simulink model "peacockElettricaSimulink"  (R2026a)
settings: Solver=FixedStepAuto  StopTime=40  FixedStep=0.001  EnableMultiTasking=on
InitFcn:
  | run('setupParams.m');
  | %run("tracks\track2.m");
StopFcn:
  | plot(out.X, out.Y);
  | axis equal;
  | grid on;
model workspace: external: MATLAB File (data not in the file)
values from neighbouring files (symbols this model uses):
  aero_bal_r = 0.5    [setupParams.m]    (also in setupParamsSingle.m)
  Af = 1.1    [setupParams.m]    (also in setupParamsSingle.m)
  auto_speed = 0    [setupParams.m]
  ay_limit = 15.0    (= 15)    [setupParams.m]    (also in setupParamsSingle.m)
  brake_bias_f = 0.40    (= 0.4)    [setupParams.m]    (also in setupParamsSingle.m = 0.6)
  brake_bias_r = 1 - brake_bias_f    (= 0.6)    [setupParams.m]    (also in setupParamsSingle.m = 0.4)
  camber_front = -1.5    [setupParams.m]    (also in setupParamsSingle.m)
  camber_rear = -1    [setupParams.m]    (also in setupParamsSingle.m)
  Cl = 1.0    (= 1)    [setupParams.m]    (also in setupParamsSingle.m)
  deathzone_APP = 5    [setupParams.m]    (also in setupParamsSingle.m)
  e_yaw_deadzone = 0.03    [setupParams.m]
  falling_slew_rate_torque = -500    [setupParams.m]    (also in setupParamsSingle.m)
  g = 9.81    [setupParams.m]    (also in setupParamsSingle.m)
  gnd_displ = 0.0    (= 0)    [setupParams.m]    (also in setupParamsSingle.m)
  h_o = 0.35    [setupParams.m]    (also in setupParamsSingle.m)
  I_charge_max = 21    [setupParams.m]
  I_discharge_max = 90    [setupParams.m]
  K_roll_rear = 0.6    [setupParams.m]    (also in setupParamsSingle.m = 0.5)
  Kus = 0.03    [setupParams.m]    (also in setupParamsSingle.m = 0)
  l_f = 0.775    [setupParams.m]    (also in setupParamsSingle.m)
  l_r = 0.775    [setupParams.m]    (also in setupParamsSingle.m)
  launch_ramp_rate = 1000.0    (= 1000)    [setupParams.m]    (also in setupParamsSingle.m)
  launch_V_thresh = 5.0    (= 5)    [setupParams.m]    (also in setupParamsSingle.m)
  mass = 320    [setupParams.m]    (also in setupParamsSingle.m = 300)
  mu = 1.5    [setupParams.m]    (also in setupParamsSingle.m)
  nominal_ramp_rate = 1000.0    (= 1000)    [setupParams.m]    (also in setupParamsSingle.m)
  overslip_factor = 1.01    [setupParams.m]    (also in setupParamsSingle.m = 1.13)
  pa_front_wheel = 82700    [setupParams.m]    (also in setupParamsSingle.m)
  pa_rear_wheel = 82700    [setupParams.m]    (also in setupParamsSingle.m)
  pedal_bp = (0:10:100)'    [setupParams.m]    (also in setupParamsSingle.m)
  pedal_map = (pedal_bp / 100) .^ pedal_alpha    [setupParams.m]    (also in setupParamsSingle.m = (pedal_bp / 100) .^ pedal_alpha.Value)
  R_wheel = 0.2032    [setupParams.m]    (also in setupParamsSingle.m)
  regen_I_cont_A = 14.0    (= 14)    [setupParams.m]    (also in setupParamsSingle.m)
  regen_I_peak_A = 21.0    (= 21)    [setupParams.m]    (also in setupParamsSingle.m)
  regen_I_peak_dur_s = 4.0    (= 4)    [setupParams.m]    (also in setupParamsSingle.m)
  regen_P_batt_max_W = 35000    [setupParams.m]    (also in setupParamsSingle.m)
  regen_pedal_thr = 5.0    (= 5)    [setupParams.m]    (also in setupParamsSingle.m = 10)
  regen_speed_crit_rpm = 1000    [setupParams.m]    (also in setupParamsSingle.m = 500)
  regen_speed_min_rpm = 4000    [setupParams.m]    (also in setupParamsSingle.m = 3000)
  regen_T_max = 9    [setupParams.m]    (also in setupParamsSingle.m = Simulink.Parameter(T_rated.Value/2))
  rho = 1.225    [setupParams.m]    (also in setupParamsSingle.m)
  rid_eff = 0.80    (= 0.8)    [setupParams.m]    (also in setupParamsSingle.m)
  rid_ratio = 15    [setupParams.m]    (also in setupParamsSingle.m)
  rising_slew_rate_torque = 100    [setupParams.m]    (also in setupParamsSingle.m)
  rpm_safe_threshold = 100    [setupParams.m]
  scale_factor_front = ones(27, 1)    [setupParams.m]    (also in setupParamsSingle.m)
  scale_factor_rear = ones(27, 1)    [setupParams.m]    (also in setupParamsSingle.m)
  slip_bc_coeff = 10    [setupParams.m]    (also in setupParamsSingle.m = Simulink.Parameter(1.5))
  slip_filt_N = 80    [setupParams.m]    (also in setupParamsSingle.m = 15)
  slip_Kd = 0.8    [setupParams.m]    (also in setupParamsSingle.m = Simulink.Parameter(5.0))
  slip_Ki = 13.0    (= 13)    [setupParams.m]    (also in setupParamsSingle.m = Simulink.Parameter(110.0))
  slip_Kp = 50.0    (= 50)    [setupParams.m]    (also in setupParamsSingle.m = Simulink.Parameter(180.0))
  slip_low_sat = 0.0    (= 0)    [setupParams.m]    (also in setupParamsSingle.m)
  slip_ref = 0.15    [setupParams.m]    (also in setupParamsSingle.m = Simulink.Parameter(0.15))
  slip_up_sat = 25    [setupParams.m]    (also in setupParamsSingle.m = 21)
  slip_V_min = 3    [setupParams.m]    (also in setupParamsSingle.m = 1)
  steer_ratio = 4.2    [pure_pursuit.m]    (also in setupParams.m; setupParamsSingle.m)
  steering_deadband = 1    [setupParams.m]
  T_headroom_k = 13.0    (= 13)    [setupParams.m]    (also in setupParamsSingle.m = Simulink.Parameter(5.0))
  T_headroom_max = 9    [setupParams.m]    (also in setupParamsSingle.m = Simulink.Parameter(5.0))
  T_peak = 20    [setupParams.m]    (also in setupParamsSingle.m = 21)
  T_rated = 9.8    [setupParams.m]    (also in setupParamsSingle.m = Simulink.Parameter(9.8))
  track_width = (track_width_r + track_width_f)/2    (= 1.2)    [setupParams.m]    (also in setupParamsSingle.m = sqrt(track_width_r^2 + track_width_f^2))
  track_width_f = 1.2    [setupParams.m]    (also in setupParamsSingle.m)
  track_width_r = 1.2    [setupParams.m]    (also in setupParamsSingle.m)
  Ts = 0.01    [setupParams.m]    (also in setupParamsSingle.m)
  tvc_bc = 17    [setupParams.m]
  tvc_D_thresh = 0.060    (= 0.06)    [setupParams.m]    (also in setupParamsSingle.m)
  tvc_D_thresh_off = 0.03    [setupParams.m]    (also in setupParamsSingle.m)
  tvc_Kd = 100    [setupParams.m]    (also in setupParamsSingle.m = Simulink.Parameter(5))
  tvc_Ki = 150    [setupParams.m]    (also in setupParamsSingle.m = Simulink.Parameter(10))
  tvc_Kp = 650    [setupParams.m]    (also in setupParamsSingle.m = Simulink.Parameter(70))
  tvc_N_filter = 25    [setupParams.m]    (also in setupParamsSingle.m = Simulink.Parameter(20))
  tvc_sat_dMz = 700    [setupParams.m]    (also in setupParamsSingle.m = Simulink.Parameter(10.0))
  tvc_throttle_on = 3.0    (= 3)    [setupParams.m]    (also in setupParamsSingle.m = Simulink.Parameter(3.0))
  tvc_tr = 5    [setupParams.m]    (also in setupParamsSingle.m = Simulink.Parameter(1.0))
  tvc_V_off = 2.0    (= 2)    [setupParams.m]    (also in setupParamsSingle.m = Simulink.Parameter(2.0))
  tvc_V_on = 4.0    (= 4)    [setupParams.m]    (also in setupParamsSingle.m = Simulink.Parameter(4.0))
  tvc_yaw_thresh = 0.08    [setupParams.m]    (also in setupParamsSingle.m)
  tvc_yaw_thresh_off = 0.04    [setupParams.m]    (also in setupParamsSingle.m)
  V_dc = 540    [setupParams.m]    (also in setupParamsSingle.m)
  w_engine = 0.005    [setupParams.m]    (also in setupParamsSingle.m)
  wheelbase = l_f + l_r    (= 1.55)    [setupParams.m]    (also in setupParamsSingle.m)
undefined symbols (not defined in the file or in its folder): V_ref, X_ref, Y_ref
libraries: simulink x74, slpidlib x8, vehdynlibtire x8, dspsigops x4, vehdynlibsteering x2, autolibshared x2, sim3dautolib x2, sim3dlib x1, robotalgslib x1
(part 3 of 6)

== system peacockElettricaSimulink/Signal Brake Builder ==
  note: TEST2
  note: TEST1
  note: TEST3
  Constant : Constant  Value=0
  Ramp1 : simulink/Sources/Ramp  slope=50  start=20  InitialOutput=0
  Ramp10 : simulink/Sources/Ramp  slope=-30  start=21  InitialOutput=0
  Ramp3 : simulink/Sources/Ramp  slope=-30  start=33.5  InitialOutput=0
  Saturation1 : Saturate  UpperLimit=50  LowerLimit=-70
  Saturation{3,5,7,11} (4 alike) : Saturate  UpperLimit=100  LowerLimit=-70
  Saturation2 : Saturate  UpperLimit=50  LowerLimit=-50
  Saturation4 : Saturate  UpperLimit=70  LowerLimit=0
  Saturation6 : Saturate  UpperLimit=100  LowerLimit=0
  Saturation8 : Saturate  UpperLimit=70  LowerLimit=0
  Step3 : Step  Time=33  FinalValue=30  SampleTime=0
  Sum1 : Sum  Inputs=|+-
  Sum2 : Sum  Inputs=|+-
  Sum3 : Sum  Inputs=|++++
  t17 : simulink/Sources/Ramp  slope=50  start=17  InitialOutput=0
  t20_2 : simulink/Sources/Ramp  slope=+50  start=20  InitialOutput=0
  t26 : simulink/Sources/Ramp  slope=50  start=26  InitialOutput=0
  t36_2 : simulink/Sources/Ramp  slope=50  start=36  InitialOutput=0
  Brake_% : Outport
  wires:
  Constant/1 -> ?
  Sum1/1 -> ?
  t17/1 -> Saturation1/1
  Saturation4/1 -> Sum3/1
  Saturation1/1 -> Sum2/1  "50%"
  Sum3/1 -> Saturation6/1
  Saturation8/1 -> Sum3/3
  Saturation6/1 -> Brake_%/1
  Ramp3/1 -> Saturation7/1
  Sum2/1 -> ?
  t26/1 -> Saturation3/1
  Saturation2/1 -> Sum2/2  "-50%"
  Saturation7/1 -> Sum3/4
  Ramp1/1 -> Saturation4/1  "80%"
  Saturation3/1 -> Sum1/1  "100%"
  t36_2/1 -> Saturation5/1
  Ramp10/1 -> Saturation11/1
  t20_2/1 -> Saturation2/1
  Saturation5/1 -> Sum1/2  "t36%"
  Saturation11/1 -> Sum3/2
  Step3/1 -> Saturation8/1  "80%"

== system peacockElettricaSimulink/Signal Brake Builder_ ==
  note: TEST2
  note: TEST1
  note: TEST3
  Constant : Constant  Value=0
  Ramp1 : simulink/Sources/Ramp  slope=50  start=20  InitialOutput=0
  Ramp10 : simulink/Sources/Ramp  slope=-30  start=21  InitialOutput=0
  Ramp3 : simulink/Sources/Ramp  slope=-30  start=33.5  InitialOutput=0
  Saturation1 : Saturate  UpperLimit=50  LowerLimit=-70
  Saturation{3,5,7,11} (4 alike) : Saturate  UpperLimit=100  LowerLimit=-70
  Saturation2 : Saturate  UpperLimit=50  LowerLimit=-50
  Saturation4 : Saturate  UpperLimit=70  LowerLimit=0
  Saturation6 : Saturate  UpperLimit=100  LowerLimit=0
  Saturation8 : Saturate  UpperLimit=70  LowerLimit=0
  Step3 : Step  Time=33  FinalValue=30  SampleTime=0
  Sum1 : Sum  Inputs=|+-
  Sum2 : Sum  Inputs=|+-
  Sum3 : Sum  Inputs=|++++
  t17 : simulink/Sources/Ramp  slope=50  start=17  InitialOutput=0
  t20_2 : simulink/Sources/Ramp  slope=+50  start=20  InitialOutput=0
  t26 : simulink/Sources/Ramp  slope=50  start=26  InitialOutput=0
  t36_2 : simulink/Sources/Ramp  slope=50  start=36  InitialOutput=0
  Brake_% : Outport
  wires:
  Constant/1 -> ?
  Sum1/1 -> ?
  t17/1 -> Saturation1/1
  Saturation4/1 -> Sum3/1
  Saturation1/1 -> Sum2/1  "50%"
  Sum3/1 -> Saturation6/1
  Saturation8/1 -> Sum3/3
  Saturation6/1 -> Brake_%/1
  Ramp3/1 -> Saturation7/1
  Sum2/1 -> ?
  t26/1 -> Saturation3/1
  Saturation2/1 -> Sum2/2  "-50%"
  Saturation7/1 -> Sum3/4
  Ramp1/1 -> Saturation4/1  "80%"
  Saturation3/1 -> Sum1/1  "100%"
  t36_2/1 -> Saturation5/1
  Ramp10/1 -> Saturation11/1
  t20_2/1 -> Saturation2/1
  Saturation5/1 -> Sum1/2  "t36%"
  Saturation11/1 -> Sum3/2
  Step3/1 -> Saturation8/1  "80%"

== system peacockElettricaSimulink/Signal Steering Builde_r ==
  note: TEST2
  note: TEST1
  Constant1 : Constant  Value=0
  Ramp : simulink/Sources/Ramp  slope=20  start=3  InitialOutput=0
  Ramp1 : simulink/Sources/Ramp  slope=-20  start=7  InitialOutput=0
  Ramp2 : simulink/Sources/Ramp  slope=-30  start=7  InitialOutput=0
  Ramp3 : simulink/Sources/Ramp  slope=20  start=11  InitialOutput=0
  Ramp4 : simulink/Sources/Ramp  slope=30  start=4  InitialOutput=0
  Ramp5 : simulink/Sources/Ramp  slope=30  start=25  InitialOutput=0
  Ramp6 : simulink/Sources/Ramp  slope=-20  start=27  InitialOutput=0
  Ramp7 : simulink/Sources/Ramp  slope=-40  start=35  InitialOutput=0
  Ramp8 : simulink/Sources/Ramp  slope=30  start=37  InitialOutput=0
  Saturation{,1..5} (6 alike) : Saturate  UpperLimit=40  LowerLimit=-40
  Saturation{8..11} (4 alike) : Saturate  UpperLimit=50  LowerLimit=-50
  Saturation6 : Saturate  UpperLimit=60  LowerLimit=-60
  Saturation7 : Saturate  UpperLimit=60  LowerLimit=-60
  Sum1 : Sum  Inputs=|++++++++
  Sum2 : Sum  Inputs=|+-+-
  t2 : simulink/Sources/Ramp  slope=20  start=2  InitialOutput=0
  t20 : simulink/Sources/Ramp  slope=-20  start=20  InitialOutput=0
  t30 : simulink/Sources/Ramp  slope=-20  start=30  InitialOutput=0
  t8 : simulink/Sources/Ramp  slope=20  start=8  InitialOutput=0
  Out1 : Outport
  wires:
  Ramp4/1 -> ?
  Constant1/1 -> ?
  Sum2/1 -> ?
  Saturation9/1 -> Sum2/2
  t30/1 -> Saturation11/1
  Ramp1/1 -> Saturation1/1
  Ramp7/1 -> Saturation6/1
  Saturation2/1 -> Sum1/3
  Saturation10/1 -> Sum2/3
  Saturation3/1 -> Sum1/4
  Ramp3/1 -> Saturation3/1
  Saturation11/1 -> Sum2/4
  Saturation7/1 -> Sum1/8
  Saturation/1 -> Sum1/1
  t2/1 -> Saturation8/1
  t20/1 -> Saturation10/1
  Ramp8/1 -> Saturation7/1
  Ramp5/1 -> Saturation4/1
  Saturation8/1 -> Sum2/1
  Saturation1/1 -> Sum1/2
  Ramp2/1 -> Saturation2/1
  t8/1 -> Saturation9/1
  Sum1/1 -> Out1/1
  Saturation5/1 -> Sum1/6
  Saturation6/1 -> Sum1/7
  Ramp/1 -> Saturation/1
  Saturation4/1 -> Sum1/5
  Ramp6/1 -> Saturation5/1

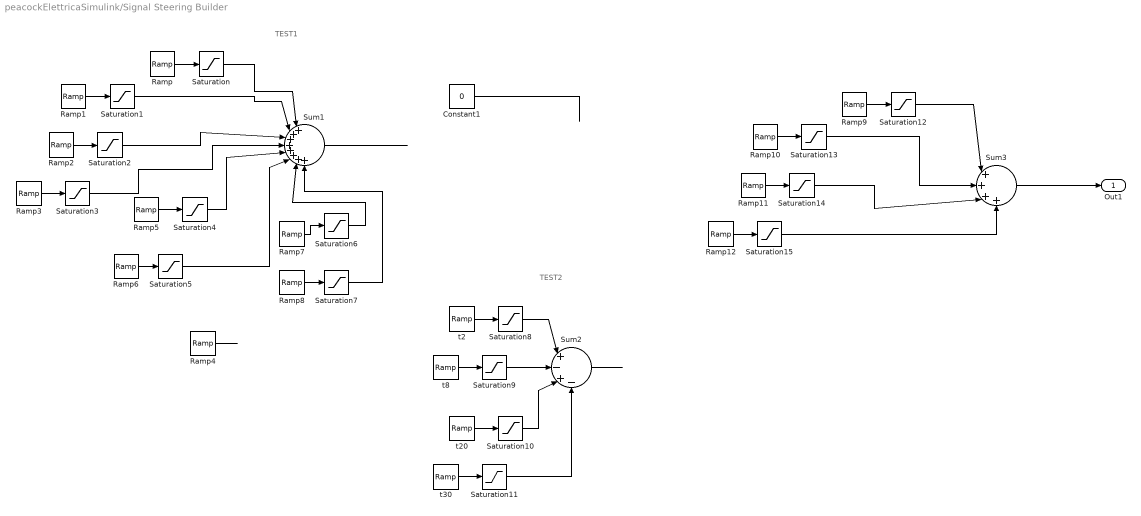
== system peacockElettricaSimulink/Signal Steering Builder ==
  note: TEST2
  note: TEST1
  Constant1 : Constant  Value=0
  Ramp : simulink/Sources/Ramp  slope=20  start=3  InitialOutput=0
  Ramp1 : simulink/Sources/Ramp  slope=-20  start=7  InitialOutput=0
  Ramp10 : simulink/Sources/Ramp  slope=-20  start=15  InitialOutput=0
  Ramp11 : simulink/Sources/Ramp  slope=-30  start=22  InitialOutput=0
  Ramp12 : simulink/Sources/Ramp  slope=30  start=27  InitialOutput=0
  Ramp2 : simulink/Sources/Ramp  slope=-30  start=7  InitialOutput=0
  Ramp3 : simulink/Sources/Ramp  slope=30  start=11  InitialOutput=0
  Ramp4 : simulink/Sources/Ramp  slope=30  start=4  InitialOutput=0
  Ramp5 : simulink/Sources/Ramp  slope=30  start=25  InitialOutput=0
  Ramp6 : simulink/Sources/Ramp  slope=-20  start=27  InitialOutput=0
  Ramp7 : simulink/Sources/Ramp  slope=-40  start=35  InitialOutput=0
  Ramp8 : simulink/Sources/Ramp  slope=30  start=37  InitialOutput=0
  Ramp9 : simulink/Sources/Ramp  slope=20  start=10  InitialOutput=0
  Saturation{,1..5,12..15} (10 alike) : Saturate  UpperLimit=40  LowerLimit=-40
  Saturation{8..11} (4 alike) : Saturate  UpperLimit=50  LowerLimit=-50
  Saturation6 : Saturate  UpperLimit=60  LowerLimit=-60
  Saturation7 : Saturate  UpperLimit=60  LowerLimit=-60
  Sum1 : Sum  Inputs=|++++++++
  Sum2 : Sum  Inputs=|+-+-
  Sum3 : Sum  Inputs=|++++
  t2 : simulink/Sources/Ramp  slope=20  start=2  InitialOutput=0
  t20 : simulink/Sources/Ramp  slope=-20  start=20  InitialOutput=0
  t30 : simulink/Sources/Ramp  slope=-20  start=30  InitialOutput=0
  t8 : simulink/Sources/Ramp  slope=20  start=8  InitialOutput=0
  Out1 : Outport
  wires:
  Ramp4/1 -> ?
  Constant1/1 -> ?
  Sum2/1 -> ?
  Saturation9/1 -> Sum2/2
  t30/1 -> Saturation11/1
  Ramp1/1 -> Saturation1/1
  Ramp7/1 -> Saturation6/1
  Saturation2/1 -> Sum1/3
  Saturation10/1 -> Sum2/3
  Saturation3/1 -> Sum1/4
  Ramp3/1 -> Saturation3/1
  Saturation11/1 -> Sum2/4
  Saturation7/1 -> Sum1/8
  Saturation/1 -> Sum1/1
  t2/1 -> Saturation8/1
  t20/1 -> Saturation10/1
  Ramp8/1 -> Saturation7/1
  Ramp5/1 -> Saturation4/1
  Saturation8/1 -> Sum2/1
  Saturation1/1 -> Sum1/2
  Ramp2/1 -> Saturation2/1
  t8/1 -> Saturation9/1
  Sum1/1 -> ?
  Saturation5/1 -> Sum1/6
  Saturation6/1 -> Sum1/7
  Ramp/1 -> Saturation/1
  Saturation4/1 -> Sum1/5
  Ramp6/1 -> Saturation5/1
  Sum3/1 -> Out1/1
  Saturation12/1 -> Sum3/1
  Saturation15/1 -> Sum3/4
  Ramp12/1 -> Saturation15/1
  Saturation13/1 -> Sum3/2
  Ramp10/1 -> Saturation13/1
  Ramp11/1 -> Saturation14/1
  Ramp9/1 -> Saturation12/1
  Saturation14/1 -> Sum3/3

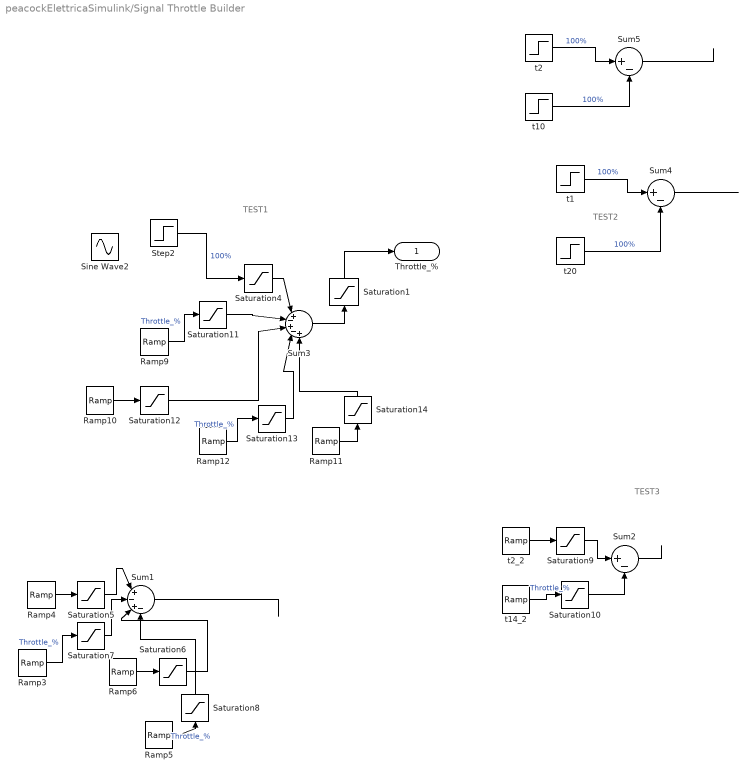
== system peacockElettricaSimulink/Signal Throttle Builder ==
  note: TEST1
  note: TEST2
  note: TEST3
  Ramp10 : simulink/Sources/Ramp  slope=50  start=26  InitialOutput=0
  Ramp11 : simulink/Sources/Ramp  slope=12  start=34  InitialOutput=0
  Ramp12 : simulink/Sources/Ramp  slope=100  start=31  InitialOutput=0
  Ramp3 : simulink/Sources/Ramp  slope=50  start=8  InitialOutput=0
  Ramp4 : simulink/Sources/Ramp  slope=150  start=1  InitialOutput=0
  Ramp5 : simulink/Sources/Ramp  slope=100  start=20  InitialOutput=0
  Ramp6 : simulink/Sources/Ramp  slope=50  start=12  InitialOutput=0
  Ramp9 : simulink/Sources/Ramp  slope=100  start=19  InitialOutput=0
  Saturation1 : Saturate  UpperLimit=50  LowerLimit=0
  Saturation{4..14} (11 alike) : Saturate  UpperLimit=100  LowerLimit=0
  Sine Wave2 : Sin  Amplitude=800  Frequency=0.3  SampleTime=Ts
  Step2 : Step  Time=2  FinalValue=100  SampleTime=0
  Sum1 : Sum  Inputs=|+-+-
  Sum2 : Sum  Inputs=|+-
  Sum3 : Sum  Inputs=|+-+-+
  Sum4 : Sum  Inputs=|+-
  Sum5 : Sum  Inputs=|+-
  t1 : Step  FinalValue=100  SampleTime=0
  t10 : Step  Time=10  FinalValue=100  SampleTime=0
  t14_2 : simulink/Sources/Ramp  slope=50  start=14  InitialOutput=0
  t2 : Step  FinalValue=100  SampleTime=0
  t20 : Step  Time=20  FinalValue=100  SampleTime=0
  t2_2 : simulink/Sources/Ramp  slope=50  start=2  InitialOutput=0
  Throttle_% : Outport
  wires:
  Sum4/1 -> ?
  Sum1/1 -> ?
  Sum2/1 -> ?
  Sum5/1 -> ?
  Step2/1 -> Saturation4/1  "100%"
  Ramp10/1 -> Saturation12/1
  Saturation7/1 -> Sum1/2
  Saturation13/1 -> Sum3/4
  Ramp9/1 -> Saturation11/1  "Throttle_%"
  t10/1 -> Sum5/2  "100%"
  Saturation5/1 -> Sum1/1
  Ramp6/1 -> Saturation6/1
  Saturation9/1 -> Sum2/1
  t2_2/1 -> Saturation9/1
  Saturation14/1 -> Sum3/5
  Saturation10/1 -> Sum2/2
  Saturation8/1 -> Sum1/4
  Saturation6/1 -> Sum1/3
  t1/1 -> Sum4/1  "100%"
  Ramp5/1 -> Saturation8/1  "Throttle_%"
  Sum3/1 -> Saturation1/1
  Ramp3/1 -> Saturation7/1  "Throttle_%"
  t20/1 -> Sum4/2  "100%"
  t2/1 -> Sum5/1  "100%"
  Ramp4/1 -> Saturation5/1
  Saturation11/1 -> Sum3/2
  Ramp12/1 -> Saturation13/1  "Throttle_%"
  Ramp11/1 -> Saturation14/1
  t14_2/1 -> Saturation10/1  "Throttle_%"
  Saturation12/1 -> Sum3/3
  Saturation4/1 -> Sum3/1
  Saturation1/1 -> Throttle_%/1

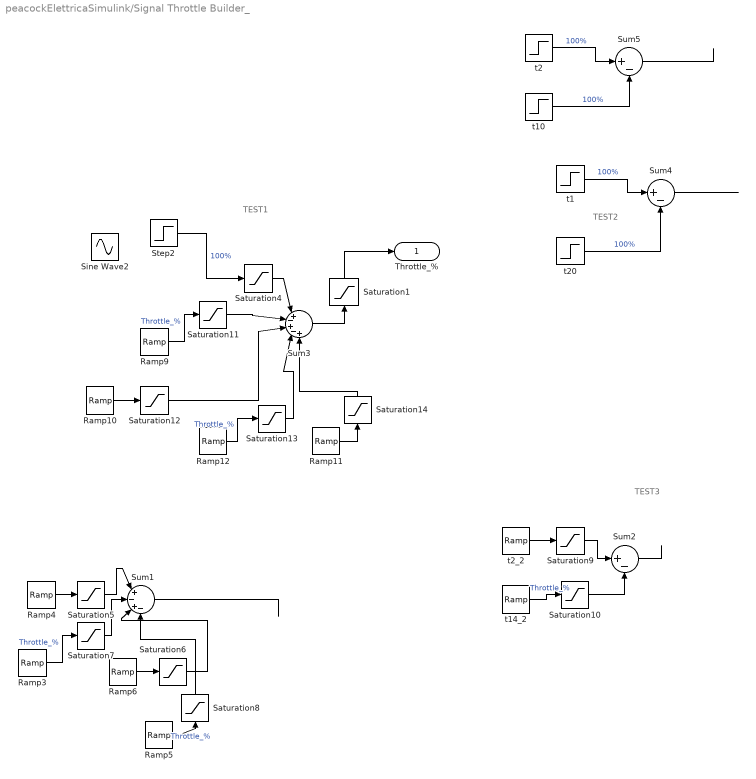
== system peacockElettricaSimulink/Signal Throttle Builder_ ==
  note: TEST1
  note: TEST2
  note: TEST3
  Ramp10 : simulink/Sources/Ramp  slope=50  start=26  InitialOutput=0
  Ramp11 : simulink/Sources/Ramp  slope=12  start=34  InitialOutput=0
  Ramp12 : simulink/Sources/Ramp  slope=100  start=31  InitialOutput=0
  Ramp3 : simulink/Sources/Ramp  slope=50  start=8  InitialOutput=0
  Ramp4 : simulink/Sources/Ramp  slope=150  start=1  InitialOutput=0
  Ramp5 : simulink/Sources/Ramp  slope=100  start=20  InitialOutput=0
  Ramp6 : simulink/Sources/Ramp  slope=50  start=12  InitialOutput=0
  Ramp9 : simulink/Sources/Ramp  slope=100  start=19  InitialOutput=0
  Saturation1 : Saturate  UpperLimit=50  LowerLimit=0
  Saturation{4..14} (11 alike) : Saturate  UpperLimit=100  LowerLimit=0
  Sine Wave2 : Sin  Amplitude=800  Frequency=0.3  SampleTime=Ts
  Step2 : Step  Time=2  FinalValue=100  SampleTime=0
  Sum1 : Sum  Inputs=|+-+-
  Sum2 : Sum  Inputs=|+-
  Sum3 : Sum  Inputs=|+-+-+
  Sum4 : Sum  Inputs=|+-
  Sum5 : Sum  Inputs=|+-
  t1 : Step  FinalValue=100  SampleTime=0
  t10 : Step  Time=10  FinalValue=100  SampleTime=0
  t14_2 : simulink/Sources/Ramp  slope=50  start=14  InitialOutput=0
  t2 : Step  FinalValue=100  SampleTime=0
  t20 : Step  Time=20  FinalValue=100  SampleTime=0
  t2_2 : simulink/Sources/Ramp  slope=50  start=2  InitialOutput=0
  Throttle_% : Outport
  wires:
  Sum4/1 -> ?
  Sum1/1 -> ?
  Sum2/1 -> ?
  Sum5/1 -> ?
  Step2/1 -> Saturation4/1  "100%"
  Ramp10/1 -> Saturation12/1
  Saturation7/1 -> Sum1/2
  Saturation13/1 -> Sum3/4
  Ramp9/1 -> Saturation11/1  "Throttle_%"
  t10/1 -> Sum5/2  "100%"
  Saturation5/1 -> Sum1/1
  Ramp6/1 -> Saturation6/1
  Saturation9/1 -> Sum2/1
  t2_2/1 -> Saturation9/1
  Saturation14/1 -> Sum3/5
  Saturation10/1 -> Sum2/2
  Saturation8/1 -> Sum1/4
  Saturation6/1 -> Sum1/3
  t1/1 -> Sum4/1  "100%"
  Ramp5/1 -> Saturation8/1  "Throttle_%"
  Sum3/1 -> Saturation1/1
  Ramp3/1 -> Saturation7/1  "Throttle_%"
  t20/1 -> Sum4/2  "100%"
  t2/1 -> Sum5/1  "100%"
  Ramp4/1 -> Saturation5/1
  Saturation11/1 -> Sum3/2
  Ramp12/1 -> Saturation13/1  "Throttle_%"
  Ramp11/1 -> Saturation14/1
  t14_2/1 -> Saturation10/1  "Throttle_%"
  Saturation12/1 -> Sum3/3
  Saturation4/1 -> Sum3/1
  Saturation1/1 -> Throttle_%/1

== system peacockElettricaSimulink/Subsystem ==
  V_ref : Inport
  V_x : Inport  Port=2
  Gain : Gain  Gain=-1
  PID Controller : slpidlib/PID Controller  Controller=PID  Form=Parallel  TimeDomain=Discrete-time  UseExternalTs=off  SampleTime=-1  IntegratorMethod=Forward Euler  FilterMethod=Forward Euler  ControllerParametersSource=internal  P=3  I=0.2  UseKiTs=off  D=0  UseExternalDerivativeSource=off  N=100  UseFilter=on  TunerSelectOption=Transfer Function Based (PID Tuner App)  InitialConditionSource=internal  InitialConditionForIntegrator=0  InitialConditionForFilter=0  DifferentiatorICPrevScaledInput=0  ExternalReset=none  TrackingMode=off  Kt=1  LimitOutput=on  SatLimitsSource=internal  UpperSaturationLimit=100  LowerSaturationLimit=-100  LinearizeAsGain=on  AntiWindupMode=clamping  Kb=1  LimitIntegrator=off  UpperIntegratorSaturationLimit=inf  LowerIntegratorSaturationLimit=-inf  POutMin=[]  POutMax=[]  IOutMin=[]  IOutMax=[]  DOutMin=[]  DOutMax=[]  NOutMin=[]  NOutMax=[]  SumOutMin=[]  SumOutMax=[]  SaturationOutMin=[]  SaturationOutMax=[]  PParamMin=[]  PParamMax=[]  IParamMin=[]  IParamMax=[]  DParamMin=[]  DParamMax=[]  NParamMin=[]  NParamMax=[]  KbParamMin=[]  KbParamMax=[]  KtParamMin=[]  KtParamMax=[]  KbOutMin=[]  KbOutMax=[]  KtOutMin=[]  KtOutMax=[]  IntegratorOutMin=[]  IntegratorOutMax=[]  FilterOutMin=[]  FilterOutMax=[]  SumI1OutMin=[]  SumI1OutMax=[]  SumI2OutMin=[]  SumI2OutMax=[]  SumI3OutMin=[]  SumI3OutMax=[]  SumI4OutMin=[]  SumI4OutMax=[]  SumDOutMin=[]  SumDOutMax=[]  DifferentiatorOutMin=[]  DifferentiatorOutMax=[]  FilterDiffOutCoefMin=[]  FilterDiffOutCoefMax=[]  ReciprocalOutMin=[]  ReciprocalOutMax=[]  SumDenOutMin=[]  SumDenOutMax=[]  SumNumOutMin=[]  SumNumOutMax=[]  DivideOutMin=[]  DivideOutMax=[]  UdiffTsProdOutMin=[]  UdiffTsProdOutMax=[]  NTsProdOutMin=[]  NTsProdOutMax=[]  UintegralTsProdOutMin=[]  UintegralTsProdOutMax=[]  UngainTsProdOutMin=[]  UngainTsProdOutMax=[]  ClampingZeroOutDataTypeStr=Inherit: Inherit via back propagation  ClampingZeroOutMin=[]  ClampingZeroOutMax=[]  FilterDenConstantOutDataTypeStr=Inherit: Inherit via back propagation  FilterDenConstantOutMin=[]  FilterDenConstantOutMax=[]  PCopyOutDataTypeStr=Inherit: Inherit via back propagation  PCopyOutMin=[]  PCopyOutMax=[]  NCopyOutDataTypeStr=Inherit: Inherit via back propagation  NCopyOutMin=[]  NCopyOutMax=[]  IntegratorContinuousStateAttributes=''  IntegratorStateMustResolveToSignalObject=off  IntegratorRTWStateStorageClass=Auto  FilterContinuousStateAttributes=''  FilterStateMustResolveToSignalObject=off  FilterRTWStateStorageClass=Auto  ParallelPVariant=InternalParameters  IdealPVariant=Disabled  IVariant=InternalParameters  DVariant=InternalParameters  IntegratorVariant=Discrete  SatVariant=Enabled  AWVariant=DiscClampingParallel  PCopyVariant=Disabled  TRVariant=Disabled  FdbkBlocksVariant=Forward  IdealPFdbkVariant=Disabled  SatFdbkVariant=Disabled  DerivativeFilterVariant=ForwardEulerFilter  NVariant=InternalParameters  NCopyVariant=Disabled  FilterICVariant=InternalICsFilter  IntegratorICVariant=InternalICs  ExternalResetVariant=Disabled  TRSumVariant=Passthrough  SumFdbkVariant=Disabled  SumVariant=Sum_PID  TsampFilterVariant=InternalTs  TsampNgainVariant=Passthrough  TsampIntegralVariant=Disabled_SignalSpec  ExternalSaturationOutDataTypeStr=Inherit: Same as second input  DerivativeSourceVariant=ErrorSignal  PreIntVariant=InternalPreInt
  Rate Limiter : RateLimiter  RisingSlewLimit=200  FallingSlewLimit=-500  SampleTimeMode=inherited
  Rate Limiter1 : RateLimiter  RisingSlewLimit=200  FallingSlewLimit=-500  SampleTimeMode=inherited
  Sum : Sum  Inputs=|+-
  brake : Saturate  UpperLimit=60  LowerLimit=0
  throttle : Saturate  UpperLimit=60  LowerLimit=0
  Throttle_% : Outport
  Brake_% : Outport  Port=2
  wires:
  PID Controller/1 -> throttle/1, Gain/1
  V_x/1 -> Sum/2
  Sum/1 -> PID Controller/1  "e_vx"
  throttle/1 -> Rate Limiter/1
  Gain/1 -> brake/1
  brake/1 -> Rate Limiter1/1
  Rate Limiter/1 -> Throttle_%/1
  Rate Limiter1/1 -> Brake_%/1
  V_ref/1 -> Sum/1

== system peacockElettricaSimulink/Subsystem1 ==
  V_x : Inport
  V_ref : Inport  Port=2
  Gain : Gain  Gain=-1
  PID Controller : slpidlib/PID Controller  Controller=PID  Form=Parallel  TimeDomain=Discrete-time  UseExternalTs=off  SampleTime=-1  IntegratorMethod=Forward Euler  FilterMethod=Forward Euler  ControllerParametersSource=internal  P=7  I=0.8  UseKiTs=off  D=1.5  UseExternalDerivativeSource=off  N=80  UseFilter=on  TunerSelectOption=Transfer Function Based (PID Tuner App)  InitialConditionSource=internal  InitialConditionForIntegrator=0  InitialConditionForFilter=0  DifferentiatorICPrevScaledInput=0  ExternalReset=none  TrackingMode=off  Kt=1  LimitOutput=on  SatLimitsSource=internal  UpperSaturationLimit=100  LowerSaturationLimit=-100  LinearizeAsGain=on  AntiWindupMode=back-calculation  Kb=2  LimitIntegrator=off  UpperIntegratorSaturationLimit=inf  LowerIntegratorSaturationLimit=-inf  POutMin=[]  POutMax=[]  IOutMin=[]  IOutMax=[]  DOutMin=[]  DOutMax=[]  NOutMin=[]  NOutMax=[]  SumOutMin=[]  SumOutMax=[]  SaturationOutMin=[]  SaturationOutMax=[]  PParamMin=[]  PParamMax=[]  IParamMin=[]  IParamMax=[]  DParamMin=[]  DParamMax=[]  NParamMin=[]  NParamMax=[]  KbParamMin=[]  KbParamMax=[]  KtParamMin=[]  KtParamMax=[]  KbOutMin=[]  KbOutMax=[]  KtOutMin=[]  KtOutMax=[]  IntegratorOutMin=[]  IntegratorOutMax=[]  FilterOutMin=[]  FilterOutMax=[]  SumI1OutMin=[]  SumI1OutMax=[]  SumI2OutMin=[]  SumI2OutMax=[]  SumI3OutMin=[]  SumI3OutMax=[]  SumI4OutMin=[]  SumI4OutMax=[]  SumDOutMin=[]  SumDOutMax=[]  DifferentiatorOutMin=[]  DifferentiatorOutMax=[]  FilterDiffOutCoefMin=[]  FilterDiffOutCoefMax=[]  ReciprocalOutMin=[]  ReciprocalOutMax=[]  SumDenOutMin=[]  SumDenOutMax=[]  SumNumOutMin=[]  SumNumOutMax=[]  DivideOutMin=[]  DivideOutMax=[]  UdiffTsProdOutMin=[]  UdiffTsProdOutMax=[]  NTsProdOutMin=[]  NTsProdOutMax=[]  UintegralTsProdOutMin=[]  UintegralTsProdOutMax=[]  UngainTsProdOutMin=[]  UngainTsProdOutMax=[]  ClampingZeroOutDataTypeStr=Inherit: Inherit via back propagation  ClampingZeroOutMin=[]  ClampingZeroOutMax=[]  FilterDenConstantOutDataTypeStr=Inherit: Inherit via back propagation  FilterDenConstantOutMin=[]  FilterDenConstantOutMax=[]  PCopyOutDataTypeStr=Inherit: Inherit via back propagation  PCopyOutMin=[]  PCopyOutMax=[]  NCopyOutDataTypeStr=Inherit: Inherit via back propagation  NCopyOutMin=[]  NCopyOutMax=[]  IntegratorContinuousStateAttributes=''  IntegratorStateMustResolveToSignalObject=off  IntegratorRTWStateStorageClass=Auto  FilterContinuousStateAttributes=''  FilterStateMustResolveToSignalObject=off  FilterRTWStateStorageClass=Auto  ParallelPVariant=InternalParameters  IdealPVariant=Disabled  IVariant=InternalParameters  DVariant=InternalParameters  IntegratorVariant=Discrete  SatVariant=Enabled  AWVariant=BackCalculation  PCopyVariant=Disabled  TRVariant=Disabled  FdbkBlocksVariant=Forward  IdealPFdbkVariant=Disabled  SatFdbkVariant=Disabled  DerivativeFilterVariant=ForwardEulerFilter  NVariant=InternalParameters  NCopyVariant=Disabled  FilterICVariant=InternalICsFilter  IntegratorICVariant=InternalICs  ExternalResetVariant=Disabled  TRSumVariant=Passthrough  SumFdbkVariant=Disabled  SumVariant=Sum_PID  TsampFilterVariant=InternalTs  TsampNgainVariant=Passthrough  TsampIntegralVariant=Disabled_SignalSpec  ExternalSaturationOutDataTypeStr=Inherit: Same as second input  DerivativeSourceVariant=ErrorSignal  PreIntVariant=InternalPreInt
  Rate Limiter : RateLimiter  RisingSlewLimit=200  FallingSlewLimit=-500  SampleTimeMode=inherited
  Rate Limiter1 : RateLimiter  RisingSlewLimit=200  FallingSlewLimit=-500  SampleTimeMode=inherited
  Sum : Sum  Inputs=|+-
  brake : Saturate  UpperLimit=60  LowerLimit=0
  throttle : Saturate  UpperLimit=100  LowerLimit=0
  Throttle_% : Outport
  Brake_% : Outport  Port=2
  wires:
  PID Controller/1 -> throttle/1, Gain/1
  V_x/1 -> Sum/2
  Sum/1 -> PID Controller/1  "e_vx"
  throttle/1 -> Rate Limiter/1
  Gain/1 -> brake/1
  brake/1 -> Rate Limiter1/1
  Rate Limiter/1 -> Throttle_%/1
  Rate Limiter1/1 -> Brake_%/1
  V_ref/1 -> Sum/1

== system peacockElettricaSimulink/DriveController/LaunchThrottleController ==
  V : Inport
  Throttle_% : Inport  Port=2
  1-D Lookup Table : Lookup_n-D  NumberOfTableDimensions=1  BreakpointsForDimension1=pedal_bp  Table=pedal_map  ExtrapMethod=Clip  UseLastTableValue=on  InternalRulePriority=Speed  RndMeth=Simplest
  Constant : Constant  Value=0
  Gain5 : Gain  Gain=100
  Rate Limiter1 : RateLimiter  RisingSlewLimit=launch_ramp_rate  FallingSlewLimit=-250  SampleTimeMode=inherited
  Rate Limiter2 : RateLimiter  RisingSlewLimit=nominal_ramp_rate  FallingSlewLimit=-250  SampleTimeMode=inherited
  Saturation : Saturate  UpperLimit=100  LowerLimit=0
  Saturation1 : Saturate  UpperLimit=100  LowerLimit=0
  Switch : Switch  Criteria=u2 > Threshold  Threshold=launch_V_thresh  SaturateOnIntegerOverflow=off  InputSameDT=off
  Switch1 : Switch  Criteria=u2 > Threshold  Threshold=deathzone_APP  SaturateOnIntegerOverflow=off  InputSameDT=off
  Throttle : Outport
  wires:
  1-D Lookup Table/1 -> Gain5/1
  Gain5/1 -> Rate Limiter1/1
  Switch1/1 -> Throttle/1  "Throttle%"
  Saturation1/1 -> Rate Limiter2/1, 1-D Lookup Table/1
  Rate Limiter2/1 -> Switch/3  "Throttle%"
  Rate Limiter1/1 -> Switch/1  "Throttle%"
  V/1 -> Switch/2
  Switch/1 -> Saturation/1  "Throttle%"
  Saturation/1 -> Switch1/1  "Throttle%"
  Constant/1 -> Switch1/3
  Throttle_%/1 -> Saturation1/1, Switch1/2

== system peacockElettricaSimulink/DriveController/MTFC ==
  note: Minimum Torque Follower Controller
      | (derating)
  Throttle : Inport
  Derating_RL : Inport  Port=2
  Derating_RR : Inport  Port=3
  Constant : Constant  Value=T_peak
  Constant1 : Constant  Value=T_rated
  Gain : Gain  Gain=T_peak*0.01
  Logical Operator : Logic  Operator=OR  AllPortsSameDT=off  OutDataTypeStr=boolean
  Min : MinMax  Inputs=2
  Rate Limiter : RateLimiter  RisingSlewLimit=250  FallingSlewLimit=-250  SampleTimeMode=inherited
  Rate Limiter1 : RateLimiter  RisingSlewLimit=250  FallingSlewLimit=-10  SampleTimeMode=inherited
  Switch : Switch  Criteria=u2 > Threshold  Threshold=0.5  SaturateOnIntegerOverflow=off  InputSameDT=off
  T_req_MTFC : Outport
  wires:
  Min/1 -> Rate Limiter1/1  "out"
  Derating_RL/1 -> Logical Operator/1
  Logical Operator/1 -> Switch/2  "or"
  Derating_RR/1 -> Logical Operator/2
  Throttle/1 -> Gain/1
  Constant1/1 -> Switch/1  "rated"
  Constant/1 -> Switch/3  "peak"
  Switch/1 -> Rate Limiter/1
  Gain/1 -> Min/1  "req"
  Rate Limiter/1 -> Min/2  "T_lim_HW"
  Rate Limiter1/1 -> T_req_MTFC/1  "T_lim_HW"

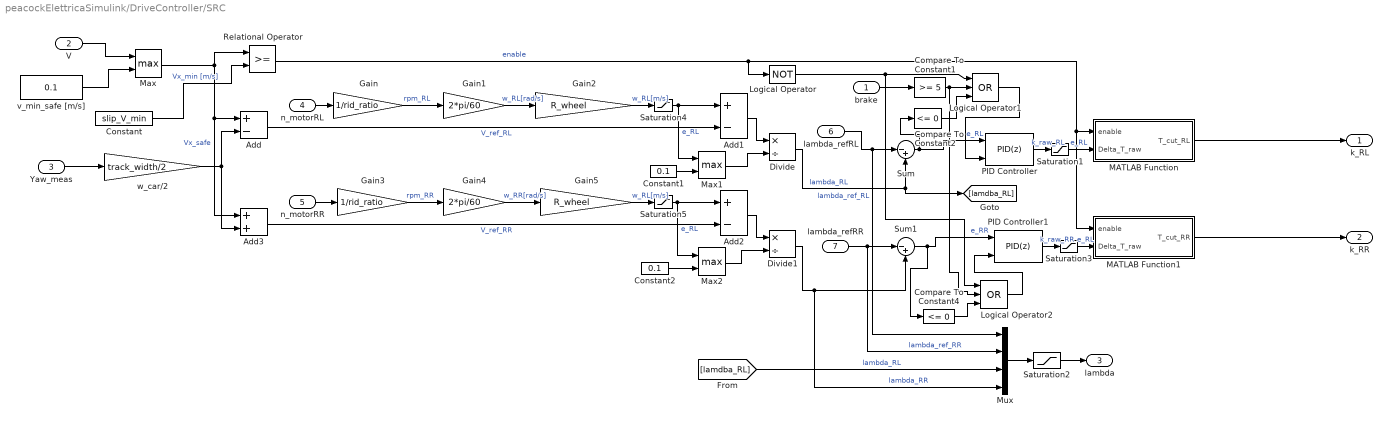
== system peacockElettricaSimulink/DriveController/SRC ==
  brake : Inport
  V : Inport  Port=2
  Yaw_meas : Inport  Port=3
  n_motorRL : Inport  Port=4
  n_motorRR : Inport  Port=5
  lambda_refRL : Inport  Port=6
  lambda_refRR : Inport  Port=7
  Add : Sum  Inputs=+-
  Add1 : Sum  Inputs=+-
  Add2 : Sum  Inputs=+-
  Add3 : Sum
  Compare To Constant1 : simulink/Logic and Bit Operations/Compare To Constant  relop=>=  const=5  OutDataTypeStr=boolean
  Compare To Constant2 : simulink/Logic and Bit Operations/Compare To Constant  relop=<=  const=0  OutDataTypeStr=boolean
  Compare To Constant4 : simulink/Logic and Bit Operations/Compare To Constant  relop=<=  const=0  OutDataTypeStr=boolean
  Constant : Constant  Value=slip_V_min
  Constant1 : Constant  Value=0.1
  Constant2 : Constant  Value=0.1
  Divide : Product  Inputs=*/
  Divide1 : Product  Inputs=*/
  Gain : Gain  Gain=1/rid_ratio
  Gain1 : Gain  Gain=2*pi/60
  Gain2 : Gain  Gain=R_wheel
  Gain3 : Gain  Gain=1/rid_ratio
  Gain4 : Gain  Gain=2*pi/60
  Gain5 : Gain  Gain=R_wheel
  Logical Operator : Logic  Operator=NOT  AllPortsSameDT=off  OutDataTypeStr=boolean
  Logical Operator1 : Logic  Operator=OR  Inputs=3  AllPortsSameDT=off  OutDataTypeStr=boolean
  Logical Operator2 : Logic  Operator=OR  Inputs=3  AllPortsSameDT=off  OutDataTypeStr=boolean
  MATLAB Function : MATLAB Function  TreatAsAtomicUnit=on
  MATLAB Function1 : MATLAB Function  TreatAsAtomicUnit=on
  Max : MinMax  Function=max  Inputs=2
  Max1 : MinMax  Function=max  Inputs=2
  Max2 : MinMax  Function=max  Inputs=2
  Mux : Mux
  PID Controller : slpidlib/PID Controller  Controller=PID  Form=Parallel  TimeDomain=Discrete-time  UseExternalTs=off  SampleTime=Ts  IntegratorMethod=Forward Euler  FilterMethod=Forward Euler  ControllerParametersSource=internal  P=slip_Kp  I=slip_Ki  UseKiTs=off  D=slip_Kd  UseExternalDerivativeSource=off  N=slip_filt_N  UseFilter=on  TunerSelectOption=Transfer Function Based (PID Tuner App)  InitialConditionSource=internal  InitialConditionForIntegrator=0  InitialConditionForFilter=0  DifferentiatorICPrevScaledInput=0  ExternalReset=level  TrackingMode=off  Kt=1  LimitOutput=on  SatLimitsSource=internal  UpperSaturationLimit=slip_up_sat  LowerSaturationLimit=slip_low_sat  LinearizeAsGain=on  AntiWindupMode=back-calculation  Kb=slip_bc_coeff  LimitIntegrator=on  UpperIntegratorSaturationLimit=slip_up_sat  LowerIntegratorSaturationLimit=slip_low_sat  POutMin=[]  POutMax=[]  IOutMin=[]  IOutMax=[]  DOutMin=[]  DOutMax=[]  NOutMin=[]  NOutMax=[]  SumOutMin=[]  SumOutMax=[]  SaturationOutMin=[]  SaturationOutMax=[]  PParamMin=[]  PParamMax=[]  IParamMin=[]  IParamMax=[]  DParamMin=[]  DParamMax=[]  NParamMin=[]  NParamMax=[]  KbParamMin=[]  KbParamMax=[]  KtParamMin=[]  KtParamMax=[]  KbOutMin=[]  KbOutMax=[]  KtOutMin=[]  KtOutMax=[]  IntegratorOutMin=[]  IntegratorOutMax=[]  FilterOutMin=[]  FilterOutMax=[]  SumI1OutMin=[]  SumI1OutMax=[]  SumI2OutMin=[]  SumI2OutMax=[]  SumI3OutMin=[]  SumI3OutMax=[]  SumI4OutMin=[]  SumI4OutMax=[]  SumDOutMin=[]  SumDOutMax=[]  DifferentiatorOutMin=[]  DifferentiatorOutMax=[]  FilterDiffOutCoefMin=[]  FilterDiffOutCoefMax=[]  ReciprocalOutMin=[]  ReciprocalOutMax=[]  SumDenOutMin=[]  SumDenOutMax=[]  SumNumOutMin=[]  SumNumOutMax=[]  DivideOutMin=[]  DivideOutMax=[]  UdiffTsProdOutMin=[]  UdiffTsProdOutMax=[]  NTsProdOutMin=[]  NTsProdOutMax=[]  UintegralTsProdOutMin=[]  UintegralTsProdOutMax=[]  UngainTsProdOutMin=[]  UngainTsProdOutMax=[]  ClampingZeroOutDataTypeStr=Inherit: Inherit via back propagation  ClampingZeroOutMin=[]  ClampingZeroOutMax=[]  FilterDenConstantOutDataTypeStr=Inherit: Inherit via back propagation  FilterDenConstantOutMin=[]  FilterDenConstantOutMax=[]  PCopyOutDataTypeStr=Inherit: Inherit via back propagation  PCopyOutMin=[]  PCopyOutMax=[]  NCopyOutDataTypeStr=Inherit: Inherit via back propagation  NCopyOutMin=[]  NCopyOutMax=[]  IntegratorContinuousStateAttributes=''  IntegratorStateMustResolveToSignalObject=off  IntegratorRTWStateStorageClass=Auto  FilterContinuousStateAttributes=''  FilterStateMustResolveToSignalObject=off  FilterRTWStateStorageClass=Auto  ParallelPVariant=InternalParameters  IdealPVariant=Disabled  IVariant=InternalParameters  DVariant=InternalParameters  IntegratorVariant=Discrete  SatVariant=Enabled  AWVariant=BackCalculation  PCopyVariant=Disabled  TRVariant=Disabled  FdbkBlocksVariant=Forward  IdealPFdbkVariant=Disabled  SatFdbkVariant=Disabled  DerivativeFilterVariant=ForwardEulerFilter  NVariant=InternalParameters  NCopyVariant=Disabled  FilterICVariant=InternalICsFilter  IntegratorICVariant=InternalICs  ExternalResetVariant=ExternalReset  TRSumVariant=Passthrough  SumFdbkVariant=Disabled  SumVariant=Sum_PID  TsampFilterVariant=InternalTs  TsampNgainVariant=Passthrough  TsampIntegralVariant=Disabled_SignalSpec  ExternalSaturationOutDataTypeStr=Inherit: Same as second input  DerivativeSourceVariant=ErrorSignal  PreIntVariant=InternalPreInt
  PID Controller1 : slpidlib/PID Controller  Controller=PID  Form=Parallel  TimeDomain=Discrete-time  UseExternalTs=off  SampleTime=Ts  IntegratorMethod=Forward Euler  FilterMethod=Forward Euler  ControllerParametersSource=internal  P=slip_Kp  I=slip_Ki  UseKiTs=off  D=slip_Kd  UseExternalDerivativeSource=off  N=slip_filt_N  UseFilter=on  TunerSelectOption=Transfer Function Based (PID Tuner App)  InitialConditionSource=internal  InitialConditionForIntegrator=0  InitialConditionForFilter=0  DifferentiatorICPrevScaledInput=0  ExternalReset=level  TrackingMode=off  Kt=1  LimitOutput=on  SatLimitsSource=internal  UpperSaturationLimit=slip_up_sat  LowerSaturationLimit=slip_low_sat  LinearizeAsGain=on  AntiWindupMode=back-calculation  Kb=slip_bc_coeff  LimitIntegrator=on  UpperIntegratorSaturationLimit=slip_up_sat  LowerIntegratorSaturationLimit=slip_low_sat  POutMin=[]  POutMax=[]  IOutMin=[]  IOutMax=[]  DOutMin=[]  DOutMax=[]  NOutMin=[]  NOutMax=[]  SumOutMin=[]  SumOutMax=[]  SaturationOutMin=[]  SaturationOutMax=[]  PParamMin=[]  PParamMax=[]  IParamMin=[]  IParamMax=[]  DParamMin=[]  DParamMax=[]  NParamMin=[]  NParamMax=[]  KbParamMin=[]  KbParamMax=[]  KtParamMin=[]  KtParamMax=[]  KbOutMin=[]  KbOutMax=[]  KtOutMin=[]  KtOutMax=[]  IntegratorOutMin=[]  IntegratorOutMax=[]  FilterOutMin=[]  FilterOutMax=[]  SumI1OutMin=[]  SumI1OutMax=[]  SumI2OutMin=[]  SumI2OutMax=[]  SumI3OutMin=[]  SumI3OutMax=[]  SumI4OutMin=[]  SumI4OutMax=[]  SumDOutMin=[]  SumDOutMax=[]  DifferentiatorOutMin=[]  DifferentiatorOutMax=[]  FilterDiffOutCoefMin=[]  FilterDiffOutCoefMax=[]  ReciprocalOutMin=[]  ReciprocalOutMax=[]  SumDenOutMin=[]  SumDenOutMax=[]  SumNumOutMin=[]  SumNumOutMax=[]  DivideOutMin=[]  DivideOutMax=[]  UdiffTsProdOutMin=[]  UdiffTsProdOutMax=[]  NTsProdOutMin=[]  NTsProdOutMax=[]  UintegralTsProdOutMin=[]  UintegralTsProdOutMax=[]  UngainTsProdOutMin=[]  UngainTsProdOutMax=[]  ClampingZeroOutDataTypeStr=Inherit: Inherit via back propagation  ClampingZeroOutMin=[]  ClampingZeroOutMax=[]  FilterDenConstantOutDataTypeStr=Inherit: Inherit via back propagation  FilterDenConstantOutMin=[]  FilterDenConstantOutMax=[]  PCopyOutDataTypeStr=Inherit: Inherit via back propagation  PCopyOutMin=[]  PCopyOutMax=[]  NCopyOutDataTypeStr=Inherit: Inherit via back propagation  NCopyOutMin=[]  NCopyOutMax=[]  IntegratorContinuousStateAttributes=''  IntegratorStateMustResolveToSignalObject=off  IntegratorRTWStateStorageClass=Auto  FilterContinuousStateAttributes=''  FilterStateMustResolveToSignalObject=off  FilterRTWStateStorageClass=Auto  ParallelPVariant=InternalParameters  IdealPVariant=Disabled  IVariant=InternalParameters  DVariant=InternalParameters  IntegratorVariant=Discrete  SatVariant=Enabled  AWVariant=BackCalculation  PCopyVariant=Disabled  TRVariant=Disabled  FdbkBlocksVariant=Forward  IdealPFdbkVariant=Disabled  SatFdbkVariant=Disabled  DerivativeFilterVariant=ForwardEulerFilter  NVariant=InternalParameters  NCopyVariant=Disabled  FilterICVariant=InternalICsFilter  IntegratorICVariant=InternalICs  ExternalResetVariant=ExternalReset  TRSumVariant=Passthrough  SumFdbkVariant=Disabled  SumVariant=Sum_PID  TsampFilterVariant=InternalTs  TsampNgainVariant=Passthrough  TsampIntegralVariant=Disabled_SignalSpec  ExternalSaturationOutDataTypeStr=Inherit: Same as second input  DerivativeSourceVariant=ErrorSignal  PreIntVariant=InternalPreInt
  Relational Operator : RelationalOperator  OutDataTypeStr=boolean  RndMeth=Simplest  InputSameDT=off
  Saturation1 : Saturate  UpperLimit=inf  LowerLimit=-2
  Saturation2 : Saturate  UpperLimit=1  LowerLimit=0
  Saturation3 : Saturate  UpperLimit=inf  LowerLimit=-2
  Saturation4 : Saturate  UpperLimit=inf  LowerLimit=0
  Saturation5 : Saturate  UpperLimit=inf  LowerLimit=0
  Sum : Sum  Inputs=|-+
  Sum1 : Sum  Inputs=|-+
  v_min_safe [m/s] : Constant  Value=0.1
  w_car/2 : Gain  Gain=track_width/2
  k_RL : Outport
  k_RR : Outport  Port=2
  lambda : Outport  Port=3
  wires:
  V/1 -> Max/1
  v_min_safe [m/s]/1 -> Max/2
  Max/1 -> Relational Operator/1, Add3/1, Add/1  "Vx_safe"
  Constant/1 -> Relational Operator/2  "Vx_min [m/s]"
  Yaw_meas/1 -> w_car/2/1
  Add/1 -> Add1/2  "V_ref_RL"
  n_motorRL/1 -> Gain/1
  Gain/1 -> Gain1/1  "rpm_RL"
  Add1/1 -> Divide/1
  Divide/1 -> [lamdba_RL], Sum/2  "lambda_RL"
  w_car/2/1 -> Add3/2, Add/2
  Gain1/1 -> Gain2/1  "w_RL[rad/s]"
  Gain2/1 -> Saturation4/1  "w_RL[m/s]"
  Gain4/1 -> Gain5/1  "w_RR[rad/s]"
  Gain3/1 -> Gain4/1  "rpm_RR"
  Divide1/1 -> Sum1/2, Mux/4  "lambda_RR"
  n_motorRR/1 -> Gain3/1
  Add3/1 -> Add2/2  "V_ref_RR"
  Add2/1 -> Divide1/1
  Relational Operator/1 -> MATLAB Function1/1(enable), MATLAB Function/1(enable), Logical Operator/1  "enable"
  PID Controller/1 -> Saturation1/1  "k_raw_RL"
  MATLAB Function/1(T_cut_RL) -> k_RL/1
  PID Controller1/1 -> Saturation3/1  "k_raw_RR"
  lambda_refRR/1 -> Mux/2, Sum1/1  "lambda_ref_RR"
  MATLAB Function1/1(T_cut_RR) -> k_RR/1
  Sum1/1 -> Compare To Constant4/1, PID Controller1/1  "e_RR"
  Sum/1 -> PID Controller/1, Compare To Constant2/1  "e_RL"
  Max1/1 -> Divide/2
  Constant1/1 -> Max1/2
  Max2/1 -> Divide1/2
  Constant2/1 -> Max2/2
  Gain5/1 -> Saturation5/1  "w_RL[m/s]"
  Mux/1 -> Saturation2/1
  Saturation2/1 -> lambda/1
  Saturation1/1 -> MATLAB Function/2(Delta_T_raw)  "e_RL"
  Saturation3/1 -> MATLAB Function1/2(Delta_T_raw)  "e_RL"
  Logical Operator1/1 -> PID Controller/2
  [lamdba_RL] -> Mux/3  "lambda_RL"
  Saturation4/1 -> Max1/1, Add1/1  "e_RL"
  Saturation5/1 -> Max2/1, Add2/1  "e_RL"
  Logical Operator/1 -> Logical Operator2/1, Logical Operator1/1
  Compare To Constant2/1 -> Logical Operator1/3
  Compare To Constant4/1 -> Logical Operator2/3
  lambda_refRL/1 -> Mux/1, Sum/1  "lambda_ref_RL"
  Logical Operator2/1 -> PID Controller1/2
  brake/1 -> Compare To Constant1/1
  Compare To Constant1/1 -> Logical Operator2/2, Logical Operator1/2

== system peacockElettricaSimulink/DriveController/TVC ==
  note: Momento Imbardata di correzione
  T_req : Inport
  e_yaw : Inport  Port=2
  T_RL_act : Inport  Port=3
  T_RR_act : Inport  Port=4
  n_motorRL : Inport  Port=5
  n_motorRR : Inport  Port=6
  D : Inport  Port=7
  w_slip : Inport  Port=8
  T_max_RL : Inport  Port=9
  T_max_RR : Inport  Port=10
  1-D Lookup Table : Lookup_n-D  NumberOfTableDimensions=1  BreakpointsForDimension1=[0,steering_deadband,4]  Table=[0,0,1]  ExtrapMethod=Clip  UseLastTableValue=on  InternalRulePriority=Speed  RndMeth=Simplest
  Abs : Abs  SaturateOnIntegerOverflow=off
  Abs1 : Abs  SaturateOnIntegerOverflow=off
  Compare To Constant : simulink/Logic and Bit Operations/Compare To Constant  relop=<=  const=0.03  OutDataTypeStr=boolean
  Constant : Constant  Value=0
  Gain : Gain  Gain=180*steer_ratio/pi
  MATLAB Function : MATLAB Function  TreatAsAtomicUnit=on
  MATLAB Function1 : MATLAB Function  TreatAsAtomicUnit=on
  Memory : Memory
  PID Controller : slpidlib/PID Controller  Controller=PID  Form=Parallel  TimeDomain=Discrete-time  UseExternalTs=off  SampleTime=Ts  IntegratorMethod=Forward Euler  FilterMethod=Forward Euler  ControllerParametersSource=internal  P=tvc_Kp  I=tvc_Ki  UseKiTs=off  D=tvc_Kd  UseExternalDerivativeSource=off  N=tvc_N_filter  UseFilter=on  TunerSelectOption=Transfer Function Based (PID Tuner App)  InitialConditionSource=internal  InitialConditionForIntegrator=0  InitialConditionForFilter=0  DifferentiatorICPrevScaledInput=0  ExternalReset=level  TrackingMode=off  Kt=tvc_tr  LimitOutput=on  SatLimitsSource=internal  UpperSaturationLimit=tvc_sat_dMz  LowerSaturationLimit=-tvc_sat_dMz  LinearizeAsGain=on  AntiWindupMode=back-calculation  Kb=tvc_bc  LimitIntegrator=off  UpperIntegratorSaturationLimit=inf  LowerIntegratorSaturationLimit=-inf  POutMin=[]  POutMax=[]  IOutMin=[]  IOutMax=[]  DOutMin=[]  DOutMax=[]  NOutMin=[]  NOutMax=[]  SumOutMin=[]  SumOutMax=[]  SaturationOutMin=[]  SaturationOutMax=[]  PParamMin=[]  PParamMax=[]  IParamMin=[]  IParamMax=[]  DParamMin=[]  DParamMax=[]  NParamMin=[]  NParamMax=[]  KbParamMin=[]  KbParamMax=[]  KtParamMin=[]  KtParamMax=[]  KbOutMin=[]  KbOutMax=[]  KtOutMin=[]  KtOutMax=[]  IntegratorOutMin=[]  IntegratorOutMax=[]  FilterOutMin=[]  FilterOutMax=[]  SumI1OutMin=[]  SumI1OutMax=[]  SumI2OutMin=[]  SumI2OutMax=[]  SumI3OutMin=[]  SumI3OutMax=[]  SumI4OutMin=[]  SumI4OutMax=[]  SumDOutMin=[]  SumDOutMax=[]  DifferentiatorOutMin=[]  DifferentiatorOutMax=[]  FilterDiffOutCoefMin=[]  FilterDiffOutCoefMax=[]  ReciprocalOutMin=[]  ReciprocalOutMax=[]  SumDenOutMin=[]  SumDenOutMax=[]  SumNumOutMin=[]  SumNumOutMax=[]  DivideOutMin=[]  DivideOutMax=[]  UdiffTsProdOutMin=[]  UdiffTsProdOutMax=[]  NTsProdOutMin=[]  NTsProdOutMax=[]  UintegralTsProdOutMin=[]  UintegralTsProdOutMax=[]  UngainTsProdOutMin=[]  UngainTsProdOutMax=[]  ClampingZeroOutDataTypeStr=Inherit: Inherit via back propagation  ClampingZeroOutMin=[]  ClampingZeroOutMax=[]  FilterDenConstantOutDataTypeStr=Inherit: Inherit via back propagation  FilterDenConstantOutMin=[]  FilterDenConstantOutMax=[]  PCopyOutDataTypeStr=Inherit: Inherit via back propagation  PCopyOutMin=[]  PCopyOutMax=[]  NCopyOutDataTypeStr=Inherit: Inherit via back propagation  NCopyOutMin=[]  NCopyOutMax=[]  IntegratorContinuousStateAttributes=''  IntegratorStateMustResolveToSignalObject=off  IntegratorRTWStateStorageClass=Auto  FilterContinuousStateAttributes=''  FilterStateMustResolveToSignalObject=off  FilterRTWStateStorageClass=Auto  ParallelPVariant=InternalParameters  IdealPVariant=Disabled  IVariant=InternalParameters  DVariant=InternalParameters  IntegratorVariant=Discrete  SatVariant=Enabled  AWVariant=BackCalculation  PCopyVariant=Disabled  TRVariant=Disabled  FdbkBlocksVariant=Forward  IdealPFdbkVariant=Disabled  SatFdbkVariant=Disabled  DerivativeFilterVariant=ForwardEulerFilter  NVariant=InternalParameters  NCopyVariant=Disabled  FilterICVariant=InternalICsFilter  IntegratorICVariant=InternalICs  ExternalResetVariant=ExternalReset  TRSumVariant=Passthrough  SumFdbkVariant=Disabled  SumVariant=Sum_PID  TsampFilterVariant=InternalTs  TsampNgainVariant=Passthrough  TsampIntegralVariant=Disabled_SignalSpec  ExternalSaturationOutDataTypeStr=Inherit: Same as second input  DerivativeSourceVariant=ErrorSignal  PreIntVariant=InternalPreInt
  Product : Product  Inputs=3
  Scope : Scope  NumInputPorts=4
      settings: ActiveDisplayYMinimum=-0.98966019020069051  ActiveDisplayYMaximum=1.1083469044144323
  Sum3 : Sum  Inputs=|-+
  TorqueAllocator : MATLAB Function  TreatAsAtomicUnit=on  SystemSampleTime=0.05
  T_TVC_RL : Outport
  T_TVC_RR : Outport  Port=2
  wires:
  PID Controller/1 -> Scope/2, MATLAB Function/1(dMz)  "dMz"
  Sum3/1 -> MATLAB Function1/1(dT_act)  "dT_act"
  MATLAB Function1/1(dMz_act) -> Memory/1  "dMz_act"
  T_RL_act/1 -> Sum3/1
  T_RR_act/1 -> Sum3/2
  Product/1 -> Scope/4, TorqueAllocator/2(dT)  "dT_real"
  TorqueAllocator/1(T_RL_cmd) -> T_TVC_RL/1
  TorqueAllocator/2(T_RR_cmd) -> T_TVC_RR/1
  n_motorRL/1 -> TorqueAllocator/3(n_motorRL)
  n_motorRR/1 -> TorqueAllocator/4(n_motorRR)
  Constant/1 -> ?
  Memory/1 -> ?
  e_yaw/1 -> PID Controller/1, Abs/1, Scope/1  "e_yaw"
  D/1 -> TorqueAllocator/5(D), Gain/1  "D_rad"
  T_req/1 -> TorqueAllocator/1(T_req)
  Gain/1 -> Abs1/1  "steering°"
  MATLAB Function/1(dT) -> Scope/3, Product/1  "dT_pi"
  1-D Lookup Table/1 -> Product/3
  Abs1/1 -> 1-D Lookup Table/1
  w_slip/1 -> Product/2
  T_max_RL/1 -> TorqueAllocator/6(T_grip_max_RL)
  T_max_RR/1 -> TorqueAllocator/7(T_grip_max_RR)
  Compare To Constant/1 -> PID Controller/2
  Abs/1 -> Compare To Constant/1

== system peacockElettricaSimulink/DriveController/Yaw_th ==
  V : Inport
  D_rad : Inport  Port=2
  Bicycle Model Dynamic : MATLAB Function  TreatAsAtomicUnit=on
  Rate Lmiter : RateLimiter  SampleTimeMode=inherited
  Trigonometric Function : Trigonometry  Operator=tan
  tand safe : MATLAB Function  TreatAsAtomicUnit=on
  yaw_saturation : MATLAB Function  TreatAsAtomicUnit=on
  yaw_th : Outport
  wires:
  tand safe/1(tand_safe) -> Bicycle Model Dynamic/2(tan_delta)  "tan delta"
  Trigonometric Function/1 -> tand safe/1(tand)
  Bicycle Model Dynamic/1(yaw_th) -> Rate Lmiter/1  "yaw_th"
  V/1 -> Bicycle Model Dynamic/1(V), yaw_saturation/2(V)  "V"
  D_rad/1 -> Trigonometric Function/1
  Rate Lmiter/1 -> yaw_saturation/1(yaw_th)  "yaw_th"
  yaw_saturation/1(yaw_sat) -> yaw_th/1  "yaw_sat"

== system peacockElettricaSimulink/DriveController_/LaunchThrottleController ==
  V : Inport
  Throttle_% : Inport  Port=2
  1-D Lookup Table : Lookup_n-D  NumberOfTableDimensions=1  BreakpointsForDimension1=pedal_bp  Table=pedal_map  ExtrapMethod=Clip  UseLastTableValue=on  InternalRulePriority=Speed  RndMeth=Simplest
  Constant : Constant  Value=0
  Gain5 : Gain  Gain=100
  Rate Limiter1 : RateLimiter  RisingSlewLimit=launch_ramp_rate  FallingSlewLimit=-250  SampleTimeMode=inherited
  Rate Limiter2 : RateLimiter  RisingSlewLimit=nominal_ramp_rate  FallingSlewLimit=-250  SampleTimeMode=inherited
  Saturation : Saturate  UpperLimit=100  LowerLimit=0
  Saturation1 : Saturate  UpperLimit=100  LowerLimit=0
  Switch : Switch  Criteria=u2 > Threshold  Threshold=launch_V_thresh  SaturateOnIntegerOverflow=off  InputSameDT=off
  Switch1 : Switch  Criteria=u2 > Threshold  Threshold=deathzone_APP  SaturateOnIntegerOverflow=off  InputSameDT=off
  Throttle : Outport
  wires:
  1-D Lookup Table/1 -> Gain5/1
  Gain5/1 -> Rate Limiter1/1
  Switch1/1 -> Throttle/1  "Throttle%"
  Saturation1/1 -> Rate Limiter2/1, 1-D Lookup Table/1
  Rate Limiter2/1 -> Switch/3  "Throttle%"
  Rate Limiter1/1 -> Switch/1  "Throttle%"
  V/1 -> Switch/2
  Switch/1 -> Saturation/1  "Throttle%"
  Saturation/1 -> Switch1/1  "Throttle%"
  Constant/1 -> Switch1/3
  Throttle_%/1 -> Saturation1/1, Switch1/2
